simulink library "commdigbbndpm2"  (Simulink 6.0)
settings: Solver=ode45  SolverMode=SingleTasking  StartTime=0.0  StopTime=10.0  RelTol=1e-3
libraries: commdigbbndpm2 x8
settings Model: RequirementInfo=9  CovMetricSettings=d  Creator=tdelve  LastModifiedBy=cvora  ExtModeAutoUpdateStatusClock=off  ProdHWDeviceType=Specified
settings DataIOCC: SignalLoggingName=logsOut
settings OptimizationCC: BooleanDataType=off
settings DebuggingCC: CheckExecutionContextPreStartOutputMsg=on  CheckExecutionContextRuntimeOutputMsg=on  SolverPrmCheckMsg=none
settings HardwareCC: ProdHWDeviceType=Specified
settings SFSimCC: SFSimApplyToAllLibs=on  SFSimBuildMode=Incremental

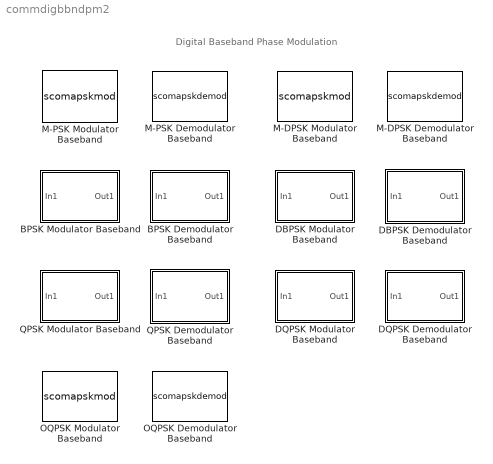
== system commdigbbndpm2 ==
  note: Digital Baseband Phase Modulation
  BPSK Demodulator Baseband : Subsystem  PropExecContextAcrossSSBoundary=on  mask(BPSK Demodulator Baseband){Ph=0, numSamp=1}
      mask prompts: Ph "Phase offset (rad):"; numSamp "Samples per symbol:"
      mask help:
      | Demodulate the input signal using the binary phase shift keying method.
      |
      | For sample-based input, the input must be a scalar. For frame-based input, the input must be a column vector.
      |
      | In case of frame-based input, the width of the input frame represents the product of the number of symbols and the Samples per symbol value.
      |
      | In case of sample-based input, the sample time of the input is the symbol period divided by the Samples per symbol value.
      mask Help: helpview(commbhelp)
      mask Display:
      | plot(0,0,100,100,[5+1.5*[[0:.8:10] [10:1.6:20] [20:.8:30]] 50 50 50 50+15*[0 1 1 2 2 3]],[85+10*[sin([0:.8:10]*pi*2/5) sin([10:1.6:20]*pi/5) sin([20:.8:30]*pi*2/5)] 85 99 75 85+8*[1 1 -1 -1 1 1]]);
      | disp('BPSK')
  BPSK Modulator Baseband : Subsystem  PropExecContextAcrossSSBoundary=on  mask(BPSK Modulator Baseband){Ph=0, numSamp=1}
      mask prompts: Ph "Phase offset (rad):"; numSamp "Samples per symbol:"
      mask help:
      | Modulate the input signal using the binary phase shift keying method.
      |
      | For sample-based input, the input must be a scalar. For frame-based input, the input must be a column vector.
      |
      | In case of frame-based input, the width of the output frame equals the product of the number of symbols and the Samples per symbol value.
      |
      | In case of sample-based input, the output sample time equals the symbol period divided by the Samples per symbol value.
      mask Help: helpview(commbhelp)
      mask Display:
      | plot(0,0,100,100,[5+15*[0 1 1 2 2 3] 50 50 50 50+1.5*[[0:.8:10] [10:1.6:20] [20:.8:30]]],[85+8*[1 1 -1 -1 1 1] 85 99 75 85+10*[sin([0:.8:10]*pi*2/5) sin([10:1.6:20]*pi/5) sin([20:.8:30]*pi*2/5)]]);
      | disp('BPSK')
  DBPSK Demodulator Baseband : Subsystem  PropExecContextAcrossSSBoundary=on  mask(DBPSK Demodulator Baseband){Ph=0, numSamp=1}
      mask prompts: Ph "Phase offset (rad):"; numSamp "Samples per symbol:"
      mask help:
      | Demodulate the input signal using the differential binary phase shift keying method.
      |
      | For sample-based input, the input must be a scalar. For frame-based input, the input must be a column vector.
      |
      | In case of frame-based input, the width of the input frame represents the product of the number of symbols and the Samples per symbol value.
      |
      | In case of sample-based input, the sample time of the input is the symbol period divided by the Samples per symbol value.
      mask Help: helpview(commbhelp)
      mask Display:
      | plot(0,0,100,100,[5+1.5*[[0:.8:10] [10:1.6:20] [20:.8:30]] 50 50 50 50+15*[0 1 1 2 2 3]],[85+10*[sin([0:.8:10]*pi*2/5) sin([10:1.6:20]*pi/5) sin([20:.8:30]*pi*2/5)] 85 99 75 85+8*[1 1 -1 -1 1 1]]);
      | disp('DBPSK')
  DBPSK Modulator Baseband : Subsystem  PropExecContextAcrossSSBoundary=on  mask(DBPSK Modulator Baseband){Ph=0, numSamp=1}
      mask prompts: Ph "Phase offset (rad):"; numSamp "Samples per symbol:"
      mask help:
      | Modulate the input signal using the differential binary phase shift keying method.
      |
      | For sample-based input, the input must be a scalar. For frame-based input, the input must be a column vector.
      |
      | In case of frame-based input, the width of the output frame equals the product of the number of symbols and the Samples per symbol value.
      |
      | In case of sample-based input, the output sample time equals the symbol period divided by the Samples per symbol value.
      mask Help: helpview(commbhelp)
      mask Display:
      | plot(0,0,100,100,[5+15*[0 1 1 2 2 3] 50 50 50 50+1.5*[[0:.8:10] [10:1.6:20] [20:.8:30]]],[85+8*[1 1 -1 -1 1 1] 85 99 75 85+10*[sin([0:.8:10]*pi*2/5) sin([10:1.6:20]*pi/5) sin([20:.8:30]*pi*2/5)]]);
      | disp('DBPSK')
  DQPSK Demodulator Baseband : Subsystem  PropExecContextAcrossSSBoundary=on  mask(DQPSK Demodulator Baseband){OutType=Integer, Dec=Binary, Ph=pi/4, numSamp=1}
      mask prompts: OutType "Output type:"; Dec "Constellation ordering:"; Ph "Phase offset (rad):"; numSamp "Samples per symbol:"
      mask help:
      | Demodulate the input signal using the differential quaternary phase shift keying method.
      |
      | For sample-based input, the input must be a scalar. For frame-based input, the input must be a column vector.
      |
      | The output can be either bits or integers. In case of bit output, the output width is an integer multiple of two.
      |
      | In case of frame-based input, the width of the input frame represents the product of the number of symbols and the Samples per symbol value.
      |
      | In case of sample-based input, the sample time of the input is the symbol period divided by the Samples per symbol value.
      mask init:
      | commblkdyampmdemod('M-DPSK Demodulator Baseband','update');
      | commblkqpskmod(gcb,'init');
      mask Help: helpview(commbhelp)
      mask StyleString: popup(Bit|Integer),popup(Binary|Gray),edit,edit
      mask CallbackString: commblkqpskmod(gcb,'InType');|||
      mask Display:
      | plot(0,0,100,100,[5+1.5*[[0:.8:10] [10:1.6:20] [20:.8:30]] 50 50 50 50+15*[0 1 1 2 2 3]],[85+10*[sin([0:.8:10]*pi*2/5) sin([10:1.6:20]*pi/5) sin([20:.8:30]*pi*2/5)] 85 99 75 85+8*[1 1 -1 -1 1 1]]);
      | disp('DQPSK')
  DQPSK Modulator Baseband : Subsystem  PropExecContextAcrossSSBoundary=on  mask(DQPSK Modulator Baseband){InType=Integer, Enc=Binary, Ph=pi/4, numSamp=1}
      mask prompts: InType "Input type:"; Enc "Constellation ordering:"; Ph "Phase offset (rad):"; numSamp "Samples per symbol:"
      mask help:
      | Modulate the input signal using the differential quaternary phase shift keying method.
      |
      | The input can be either bits or integers. In case of sample-based bit input, the input width must be two. In case of frame-based bit input, the input width must be an integer multiple of two. The bits can be either binary-mapped or Gray-mapped into symbols.
      |
      | For sample-based integer input, the input must be a scalar. For frame-based integer input, the input must be a column vector.
      |
      | In case of frame-based input, the width of the output frame equals the product of the number of symbols and the Samples per symbol value.
      |
      | In case of sample-based input, the output sample time equals the symbol period divided by the Samples per symbol value.
      mask init:
      | commblkdyampmmod('M-DPSK Modulator Baseband','update')
      | commblkqpskmod(gcb,'init');
      mask Help: helpview(commbhelp)
      mask StyleString: popup(Bit|Integer),popup(Binary|Gray),edit,edit
      mask CallbackString: commblkqpskmod(gcb,'InType');|||
      mask Display:
      | plot(0,0,100,100,[5+15*[0 1 1 2 2 3] 50 50 50 50+1.5*[[0:.8:10] [10:1.6:20] [20:.8:30]]],[85+8*[1 1 -1 -1 1 1] 85 99 75 85+10*[sin([0:.8:10]*pi*2/5) sin([10:1.6:20]*pi/5) sin([20:.8:30]*pi*2/5)]]);
      | disp('DQPSK')
  M-DPSK Demodulator Baseband : S-Function  FunctionName=scomapskdemod  Parameters=M,OutType,Dec,1,1,1,1,Ph,numSamp,0,0,2  mask(M-DPSK Demodulator Baseband){M=8, OutType=Integer, Dec=Binary, Ph=pi/8, numSamp=1}
      mask prompts: M "M-ary number:"; OutType "Output type:"; Dec "Constellation ordering:"; Ph "Phase offset (rad):"; numSamp "Samples per symbol:"
      mask help:
      | Demodulate the input signal using the differential phase shift keying method.
      |
      | For sample-based input, the input must be a scalar. For frame-based input, the input must be a column vector.
      |
      | The output can be either bits or integers. In case of bit output, the output width is an integer multiple of the number of bits per symbol. The symbols can be either binary-demapped or Gray-demapped into bits.
      |
      | In case of frame-based input, the width of the input frame represents the product of the number of symbols and the Samples per symbol value.
      |
      | In case of sample-based input, the sample time of the input is the symbol period divided by the Samples per symbol value.
      mask init:
      | commblkpskmod(gcb,'init');
      mask Help: helpview(commbhelp)
      mask StyleString: edit,popup(Bit|Integer),popup(Binary|Gray),edit,edit
      mask CallbackString: |commblkpskmod(gcb,'InType');|||
      mask Display:
      | plot(0,0,100,100,[5+1.5*[[0:.8:10] [10:1.6:20] [20:.8:30]] 50 50 50 50+15*[0 1 1 2 2 3]],[85+10*[sin([0:.8:10]*pi*2/5) sin([10:1.6:20]*pi/5) sin([20:.8:30]*pi*2/5)] 85 99 75 85+8*[1 1 -1 -1 1 1]]);
      | disp('M-DPSK')
  M-DPSK Modulator Baseband : S-Function  FunctionName=scomapskmod  Parameters=M,InType,Enc,1,1,1,1,Ph,numSamp,0,0,2  mask(M-DPSK Modulator Baseband){M=8, InType=Integer, Enc=Binary, Ph=pi/8, numSamp=1}
      mask prompts: M "M-ary number:"; InType "Input type:"; Enc "Constellation ordering:"; Ph "Phase offset (rad):"; numSamp "Samples per symbol:"
      mask help:
      | Modulate the input signal using the differential phase shift keying method.
      |
      | The input can be either bits or integers. In case of sample-based bit input, the input width must equal the number of bits per symbol. In case of frame-based bit input, the input width must be an integer multiple of the number of bits per symbol. The bits can be either binary-mapped or Gray-mapped into symbols.
      |
      | For sample-based integer input, the input must be a scalar. For frame-based integer input, the input must be a column vector.
      |
      | In case of frame-based input, the width of the output frame equals the product of the number of symbols and the Samples per symbol value.
      |
      | In case of sample-based input, the output sample time equals the symbol period divided by the Samples per symbol value.
      mask init:
      | commblkpskmod(gcb,'init');
      mask Help: helpview(commbhelp)
      mask StyleString: edit,popup(Bit|Integer),popup(Binary|Gray),edit,edit
      mask CallbackString: |commblkpskmod(gcb,'InType');|||
      mask Display:
      | plot(0,0,100,100,[5+15*[0 1 1 2 2 3] 50 50 50 50+1.5*[[0:.8:10] [10:1.6:20] [20:.8:30]]],[85+8*[1 1 -1 -1 1 1] 85 99 75 85+10*[sin([0:.8:10]*pi*2/5) sin([10:1.6:20]*pi/5) sin([20:.8:30]*pi*2/5)]]);
      | disp('M-DPSK')
  M-PSK Demodulator Baseband : S-Function  FunctionName=scomapskdemod  Parameters=M,OutType,Dec,1,1,1,1,Ph,numSamp,0,0,1  mask(M-PSK Demodulator Baseband){M=8, OutType=Integer, Dec=Binary, Ph=pi/8, numSamp=1}
      mask prompts: M "M-ary number:"; OutType "Output type:"; Dec "Constellation ordering:"; Ph "Phase offset (rad):"; numSamp "Samples per symbol:"
      mask help:
      | Demodulate the input signal using the phase shift keying method.
      |
      | For sample-based input, the input must be a scalar. For frame-based input, the input must be a column vector.
      |
      | The output can be either bits or integers. In case of bit output, the output width is an integer multiple of the number of bits per symbol. The symbols can be either binary-demapped or Gray-demapped into bits.
      |
      | In case of frame-based input, the width of the input frame represents the product of the number of symbols and the Samples per symbol value.
      |
      | In case of sample-based input, the sample time of the input is the symbol period divided by the Samples per symbol value.
      mask init:
      | commblkpskmod(gcb,'init');
      mask Help: helpview(commbhelp)
      mask StyleString: edit,popup(Bit|Integer),popup(Binary|Gray),edit,edit
      mask CallbackString: |commblkpskmod(gcb,'InType');|||
      mask Display:
      | plot(0,0,100,100,[5+1.5*[[0:.8:10] [10:1.6:20] [20:.8:30]] 50 50 50 50+15*[0 1 1 2 2 3]],[85+10*[sin([0:.8:10]*pi*2/5) sin([10:1.6:20]*pi/5) sin([20:.8:30]*pi*2/5)] 85 99 75 85+8*[1 1 -1 -1 1 1]]);
      | disp('M-PSK')
  M-PSK Modulator Baseband : S-Function  FunctionName=scomapskmod  Parameters=M,InType,Enc,1,1,1,1,Ph,numSamp,0,0,1  mask(M-PSK Modulator Baseband){M=8, InType=Integer, Enc=Binary, Ph=pi/8, numSamp=1}
      mask prompts: M "M-ary number:"; InType "Input type:"; Enc "Constellation ordering:"; Ph "Phase offset (rad):"; numSamp "Samples per symbol:"
      mask help:
      | Modulate the input signal using the phase shift keying method.
      |
      | The input can be either bits or integers. In case of sample-based bit input, the input width must equal the number of bits per symbol. In case of frame-based bit input, the input width must be an integer multiple of the number of bits per symbol. The bits can be either binary-mapped or Gray-mapped into symbols.
      |
      | For sample-based integer input, the input must be a scalar. For frame-based integer input, the input must be a column vector.
      |
      | In case of frame-based input, the width of the output frame equals the product of the number of symbols and the Samples per symbol value.
      |
      | In case of sample-based input, the output sample time equals the symbol period divided by the Samples per symbol value.
      mask init:
      | commblkpskmod(gcb,'init');
      mask Help: helpview(commbhelp)
      mask StyleString: edit,popup(Bit|Integer),popup(Binary|Gray),edit,edit
      mask CallbackString: |commblkpskmod(gcb,'InType');|||
      mask Display:
      | plot(0,0,100,100,[5+15*[0 1 1 2 2 3] 50 50 50 50+1.5*[[0:.8:10] [10:1.6:20] [20:.8:30]]],[85+8*[1 1 -1 -1 1 1] 85 99 75 85+10*[sin([0:.8:10]*pi*2/5) sin([10:1.6:20]*pi/5) sin([20:.8:30]*pi*2/5)]]);
      | disp('M-PSK')
  OQPSK Demodulator Baseband : S-Function  FunctionName=scomapskdemod  Parameters=4,OutType,1,1,1,1,1,Ph,numSamp,0,0,6  mask(OQPSK Demodulator Baseband){OutType=Integer, Ph=0, numSamp=1}
      mask prompts: OutType "Output type:"; Ph "Phase offset (rad):"; numSamp "Oversampling factor:"
      mask help:
      | Demodulate the input signal using the offset quadrature phase shift keying method.
      |
      | For sample-based input, the input must be a scalar. For frame-based input, the input must be a column vector.
      |
      | The output can be either bits or integers. In case of bit output, the output width is an integer multiple of two.
      |
      | In case of frame-based input, the width of the input frame represents the product of the number of symbols and twice the Oversampling factor value.
      |
      | In case of sample-based input, the sample time of the input is the symbol period divided by twice the Oversampling factor value.
      mask Help: helpview(commbhelp)
      mask StyleString: popup(Bit|Integer),edit,edit
      mask Display:
      | plot(0,0,100,100,[5+1.5*[[0:.8:10] [10:1.6:20] [20:.8:30]] 50 50 50 50+15*[0 1 1 2 2 3]],[85+10*[sin([0:.8:10]*pi*2/5) sin([10:1.6:20]*pi/5) sin([20:.8:30]*pi*2/5)] 85 99 75 85+8*[1 1 -1 -1 1 1]]);
      | disp('OQPSK')
  OQPSK Modulator Baseband : S-Function  FunctionName=scomapskmod  Parameters=4,InType,1,1,1,1,1,Ph,numSamp,0,0,6  mask(OQPSK Modulator Baseband){InType=Integer, Ph=0, numSamp=1}
      mask prompts: InType "Input type:"; Ph "Phase offset (rad):"; numSamp "Oversampling factor:"
      mask help:
      | Modulate the input signal using the offset quadrature phase shift keying method.
      |
      | The input can be either bits or integers. In case of sample-based bit input, the input width must be two. In case of frame-based bit inputs, the input width must be an integer multiple of two.
      |
      | For sample-based integer input, the input must be a scalar. For frame-based integer input, the input must be a column vector.
      |
      | In case of frame-based input, the width of the output frame equals two times the Oversampling factor value times the number of symbols.
      |
      | In case of sample-based input, the output sample time equals the symbol period divided by twice the Oversampling factor value.
      mask Help: helpview(commbhelp)
      mask StyleString: popup(Bit|Integer),edit,edit
      mask Display:
      | plot(0,0,100,100,[5+15*[0 1 1 2 2 3] 50 50 50 50+1.5*[[0:.8:10] [10:1.6:20] [20:.8:30]]],[85+8*[1 1 -1 -1 1 1] 85 99 75 85+10*[sin([0:.8:10]*pi*2/5) sin([10:1.6:20]*pi/5) sin([20:.8:30]*pi*2/5)]]);
      | disp('OQPSK')
  QPSK Demodulator Baseband : Subsystem  PropExecContextAcrossSSBoundary=on  mask(QPSK Demodulator Baseband){OutType=Integer, Dec=Binary, Ph=pi/4, numSamp=1}
      mask prompts: OutType "Output type:"; Dec "Constellation ordering:"; Ph "Phase offset (rad):"; numSamp "Samples per symbol:"
      mask help:
      | Demodulate the input signal using the quaternary phase shift keying method.
      |
      | For sample-based input, the input must be a scalar. For frame-based input, the input must be a column vector.
      |
      | The output can be either bits or integers. In case of bit output, the output width is an integer multiple of two.
      |
      | In case of frame-based input, the width of the input frame represents the product of the number of symbols and the Samples per symbol value.
      |
      | In case of sample-based input, the sample time of the input is the symbol period divided by the Samples per symbol value.
      mask init:
      | commblkdyampmdemod('M-PSK Demodulator Baseband','update');
      | commblkqpskmod(gcb,'init');
      mask Help: helpview(commbhelp)
      mask StyleString: popup(Bit|Integer),popup(Binary|Gray),edit,edit
      mask CallbackString: commblkqpskmod(gcb,'InType');|||
      mask Display:
      | plot(0,0,100,100,[5+1.5*[[0:.8:10] [10:1.6:20] [20:.8:30]] 50 50 50 50+15*[0 1 1 2 2 3]],[85+10*[sin([0:.8:10]*pi*2/5) sin([10:1.6:20]*pi/5) sin([20:.8:30]*pi*2/5)] 85 99 75 85+8*[1 1 -1 -1 1 1]]);
      | disp('QPSK')
  QPSK Modulator Baseband : Subsystem  PropExecContextAcrossSSBoundary=on  mask(QPSK Modulator Baseband){InType=Integer, Enc=Binary, Ph=pi/4, numSamp=1}
      mask prompts: InType "Input type:"; Enc "Constellation ordering:"; Ph "Phase offset (rad):"; numSamp "Samples per symbol:"
      mask help:
      | Modulate the input signal using the quaternary phase shift keying method.
      |
      | The input can be either bits or integers. In case of sample-based bit input, the input width must be two. In case of frame-based bit input, the input width must be an integer multiple of two. The bits can be either binary-mapped or Gray-mapped into symbols.
      |
      | For sample-based integer input, the input must be a scalar. For frame-based integer input, the input must be a column vector.
      |
      | In case of frame-based input, the width of the output frame equals the product of the number of symbols and the Samples per symbol value.
      |
      | In case of sample-based input, the output sample time equals the symbol period divided by the Samples per symbol value.
      mask init:
      | commblkqpskmod(gcb,'init');
      | commblkdyampmmod('M-PSK Modulator Baseband','update')
      mask Help: helpview(commbhelp)
      mask StyleString: popup(Bit|Integer),popup(Binary|Gray),edit,edit
      mask CallbackString: commblkqpskmod(gcb,'InType');|||
      mask Display:
      | plot(0,0,100,100,[5+15*[0 1 1 2 2 3] 50 50 50 50+1.5*[[0:.8:10] [10:1.6:20] [20:.8:30]]],[85+8*[1 1 -1 -1 1 1] 85 99 75 85+10*[sin([0:.8:10]*pi*2/5) sin([10:1.6:20]*pi/5) sin([20:.8:30]*pi*2/5)]]);
      | disp('QPSK')

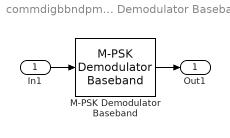
== system commdigbbndpm2/BPSK Demodulator Baseband ==
  In1 : Inport  LatchInput=off
  M-PSK Demodulator Baseband : commdigbbndpm2/M-PSK Demodulator Baseband  M=2  OutType=Integer  Dec=Binary  Ph=Ph  numSamp=numSamp
  Out1 : Outport
  wires:
  M-PSK Demodulator Baseband/1 -> Out1/1
  In1/1 -> M-PSK Demodulator Baseband/1

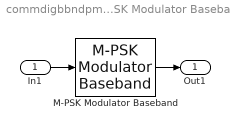
== system commdigbbndpm2/BPSK Modulator Baseband ==
  In1 : Inport  LatchInput=off
  M-PSK Modulator Baseband : commdigbbndpm2/M-PSK Modulator Baseband  M=2  InType=Integer  Enc=Binary  Ph=Ph  numSamp=numSamp
  Out1 : Outport
  wires:
  M-PSK Modulator Baseband/1 -> Out1/1
  In1/1 -> M-PSK Modulator Baseband/1

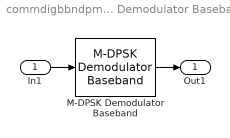
== system commdigbbndpm2/DBPSK Demodulator Baseband ==
  In1 : Inport  LatchInput=off
  M-DPSK Demodulator Baseband : commdigbbndpm2/M-DPSK Demodulator Baseband  M=2  OutType=Integer  Dec=Binary  Ph=Ph  numSamp=numSamp
  Out1 : Outport
  wires:
  M-DPSK Demodulator Baseband/1 -> Out1/1
  In1/1 -> M-DPSK Demodulator Baseband/1

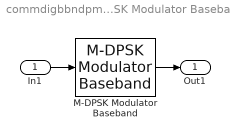
== system commdigbbndpm2/DBPSK Modulator Baseband ==
  In1 : Inport  LatchInput=off
  M-DPSK Modulator Baseband : commdigbbndpm2/M-DPSK Modulator Baseband  M=2  InType=Integer  Enc=Binary  Ph=Ph  numSamp=numSamp
  Out1 : Outport
  wires:
  M-DPSK Modulator Baseband/1 -> Out1/1
  In1/1 -> M-DPSK Modulator Baseband/1

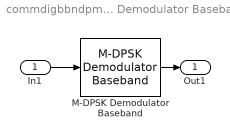
== system commdigbbndpm2/DQPSK Demodulator Baseband ==
  In1 : Inport  LatchInput=off
  M-DPSK Demodulator Baseband : commdigbbndpm2/M-DPSK Demodulator Baseband  M=4  OutType=Integer  Dec=Binary  Ph=Ph  numSamp=numSamp
  Out1 : Outport
  wires:
  M-DPSK Demodulator Baseband/1 -> Out1/1
  In1/1 -> M-DPSK Demodulator Baseband/1

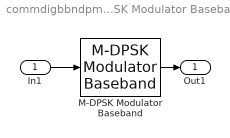
== system commdigbbndpm2/DQPSK Modulator Baseband ==
  In1 : Inport  LatchInput=off
  M-DPSK Modulator Baseband : commdigbbndpm2/M-DPSK Modulator Baseband  M=4  InType=Integer  Enc=Binary  Ph=Ph  numSamp=numSamp
  Out1 : Outport
  wires:
  M-DPSK Modulator Baseband/1 -> Out1/1
  In1/1 -> M-DPSK Modulator Baseband/1

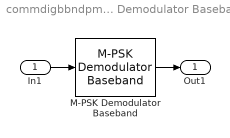
== system commdigbbndpm2/QPSK Demodulator Baseband ==
  In1 : Inport  LatchInput=off
  M-PSK Demodulator Baseband : commdigbbndpm2/M-PSK Demodulator Baseband  M=4  OutType=Integer  Dec=Binary  Ph=Ph  numSamp=numSamp
  Out1 : Outport
  wires:
  M-PSK Demodulator Baseband/1 -> Out1/1
  In1/1 -> M-PSK Demodulator Baseband/1

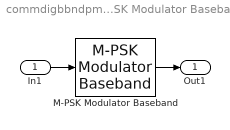
== system commdigbbndpm2/QPSK Modulator Baseband ==
  In1 : Inport  LatchInput=off
  M-PSK Modulator Baseband : commdigbbndpm2/M-PSK Modulator Baseband  M=4  InType=Integer  Enc=Binary  Ph=Ph  numSamp=numSamp
  Out1 : Outport
  wires:
  M-PSK Modulator Baseband/1 -> Out1/1
  In1/1 -> M-PSK Modulator Baseband/1
